simulink model "EE_Lab4"  (R2024b)
settings: Solver=VariableStepAuto  StartTime=0.0  StopTime=0.04  RelTol=1e-3
undefined symbols (not defined in the file): Angle, Magnitude
libraries: spsSeriesRLCBranchLib x4, spsCurrentMeasurementLib x4, spsVoltageMeasurementLib x4, spsACVoltageSourceLib x2, spsLinearTransformerLib x2, sps_lib x1, spspowerguiLib x1
settings Model: Creator=offic  LastModifiedBy=offic

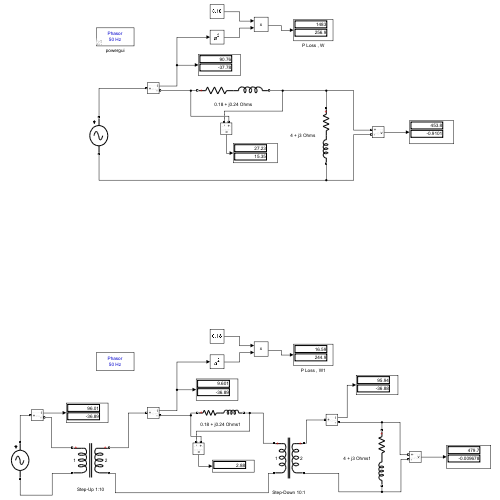
[thumbnail: Simulink's stored preview of the top-level diagram]
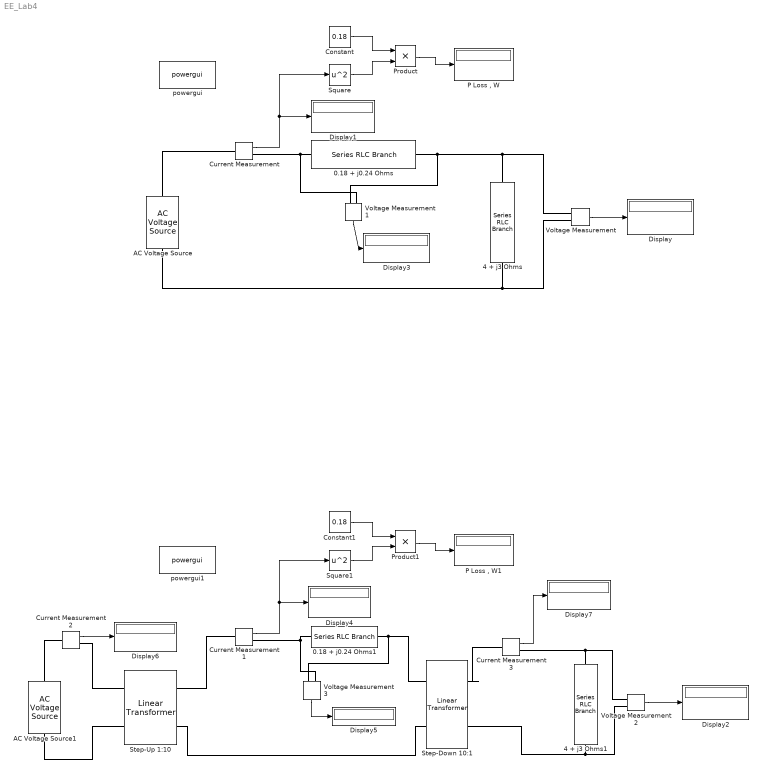
== system EE_Lab4 ==
  0.18 + j0.24 Ohms : spsSeriesRLCBranchLib/Series RLC Branch  LConnTagsString=__new0  RConnTagsString=__new0  BranchType=RL  Resistance=0.18  Inductance=0.0007639437  SetiL0=off  InitialCurrent=0  Capacitance=1e-6  Setx0=off  InitialVoltage=0  Measurements=None
  0.18 + j0.24 Ohms1 : spsSeriesRLCBranchLib/Series RLC Branch  LConnTagsString=__new0  RConnTagsString=__new0  BranchType=RL  Resistance=0.18  Inductance=0.0007639437  SetiL0=off  InitialCurrent=0  Capacitance=1e-6  Setx0=off  InitialVoltage=0  Measurements=None
  4 + j3 Ohms : spsSeriesRLCBranchLib/Series RLC Branch  LConnTagsString=__new0  RConnTagsString=__new0  BranchType=RL  Resistance=4  Inductance=0.00954929  SetiL0=off  InitialCurrent=0  Capacitance=1e-6  Setx0=off  InitialVoltage=0  Measurements=None
  4 + j3 Ohms1 : spsSeriesRLCBranchLib/Series RLC Branch  LConnTagsString=__new0  RConnTagsString=__new0  BranchType=RL  Resistance=4  Inductance=0.00954929  SetiL0=off  InitialCurrent=0  Capacitance=1e-6  Setx0=off  InitialVoltage=0  Measurements=None
  AC Voltage Source : spsACVoltageSourceLib/AC Voltage Source  Amplitude=480  Phase=0  Frequency=50  SampleTime=0  Measurements=None  BusType=swing  Pref=10e3  Qref=0  Qmin=-inf  Qmax=+inf
  AC Voltage Source1 : spsACVoltageSourceLib/AC Voltage Source  Amplitude=480  Phase=0  Frequency=50  SampleTime=0  Measurements=None  BusType=swing  Pref=10e3  Qref=0  Qmin=-inf  Qmax=+inf
  Constant : Constant  Value=0.18
  Constant1 : Constant  Value=0.18
  Current Measurement{,1..3} (4 alike) : spsCurrentMeasurementLib/Current Measurement  PhasorSimulation=on  OutputType=Magnitude-Angle  PSBequivalent=0
  Display{,1..7} (8 alike) : Display
  "P Loss , W" : Display
  "P Loss , W1" : Display
  Product : Product
  Product1 : Product
  Square : Math  Operator=square
  Square1 : Math  Operator=square
  Step-Down 10:1 : spsLinearTransformerLib/Linear Transformer  UNITS=SI  NominalPower=[ 250e6 50 ]  winding1="[ 4800  0.0000001  0.00000001]"  winding2="[ 480  0.0000001  0.00000001]"  ThreeWindings=off  winding3=[3.15e+05 0.7938 0.10107]  RmLm=[1.08e6 2866]  Measurements=None  DataType=on
  Step-Up 1:10 : spsLinearTransformerLib/Linear Transformer  UNITS=SI  NominalPower=[ 250e6 50 ]  winding1="[ 480  0.0000001  0.00000001]"  winding2="[ 4800  0.0000001  0.00000001]"  ThreeWindings=off  winding3=[3.15e+05 0.7938 0.10107]  RmLm=[1.08e6 2866]  Measurements=None  DataType=on
  Voltage Measurement : spsVoltageMeasurementLib/Voltage Measurement  PhasorSimulation=on  OutputType=Magnitude-Angle  PSBequivalent=0
  Voltage Measurement1 : spsVoltageMeasurementLib/Voltage Measurement  PhasorSimulation=on  OutputType=Magnitude-Angle  PSBequivalent=0
  Voltage Measurement2 : spsVoltageMeasurementLib/Voltage Measurement  PhasorSimulation=on  OutputType=Magnitude-Angle  PSBequivalent=0
  Voltage Measurement3 : spsVoltageMeasurementLib/Voltage Measurement  PhasorSimulation=on  OutputType=Magnitude  PSBequivalent=0
  powergui : sps_lib/powergui  Priority=1  SimulationMode=Phasor  SampleTime=50e-6  frequency=50  Iterations=50  frequencyindice=50  Pbase=100e6  ErrMax=1e-4  UnitsV=kV  UnitsW=MW  buscounter=0  FunctionMessages=off  echomessages=off  EnableUseOfTLC=off  CurrentSourceSwitches=off  DisableSnubberDevices=off  DisableRonSwitches=off  DisableVfSwitches=off  DisplayEquations=off  AutomaticDiscreteSolvers=off  SolverType=Tustin/Backward Euler (TBE)  Interpol=off  ExternalGateDelay=off  methode=off  Ts=100  x0status=blocks  SPID=on  SwTol=0  HookPort=off  NonlinearTolerance=1e-4  nMaxIteration=100  ContinueOnMaxIteration=off  RestoreLinks=warning  ResistiveCurrentMeasurement=off  Frange=[0:2:500]  Ylog=off  Xlog=on  ShowGrid=off  save=off  variable=ZData  structure=0  ZoomFFT=off  StartTime=0.0  cycles=1  DisplayStyle=1  fundamental=60  FreqAxis=off  MaxFrequency=1000  frequencyindicesteady=1  RmsSteady=1  display=off
  powergui1 : spspowerguiLib/powergui  Priority=1  SimulationMode=Phasor  SampleTime=50e-6  frequency=50  Iterations=50  frequencyindice=50  Pbase=100e6  ErrMax=1e-4  UnitsV=kV  UnitsW=MW  buscounter=0  FunctionMessages=off  echomessages=off  EnableUseOfTLC=off  CurrentSourceSwitches=off  DisableSnubberDevices=off  DisableRonSwitches=off  DisableVfSwitches=off  DisplayEquations=off  AutomaticDiscreteSolvers=off  SolverType=Tustin/Backward Euler (TBE)  Interpol=off  ExternalGateDelay=off  methode=off  Ts=100  x0status=blocks  SPID=on  SwTol=0  HookPort=off  NonlinearTolerance=1e-4  nMaxIteration=100  ContinueOnMaxIteration=off  RestoreLinks=warning  ResistiveCurrentMeasurement=off  Frange=[0:2:500]  Ylog=off  Xlog=on  ShowGrid=off  save=off  variable=ZData  structure=0  ZoomFFT=off  StartTime=0.0  cycles=1  DisplayStyle=1  fundamental=60  FreqAxis=off  MaxFrequency=1000  frequencyindicesteady=1  RmsSteady=1  display=off
  wires:
  Voltage Measurement/1 -> Display/1
  Current Measurement/1 -> Square/1, Display1/1
  Constant/1 -> Product/1
  Square/1 -> Product/2
  Product/1 -> "P Loss , W"/1
  Voltage Measurement1/1 -> Display3/1
  Voltage Measurement3/1 -> Display5/1
  Voltage Measurement2/1 -> Display2/1
  Square1/1 -> Product1/2
  Product1/1 -> "P Loss , W1"/1
  Constant1/1 -> Product1/1
  Current Measurement1/1 -> Square1/1, Display4/1
  Current Measurement2/1 -> Display6/1
  Current Measurement3/1 -> Display7/1
  connections:
  AC Voltage Source/RConn1 -- Current Measurement/LConn1
  0.18 + j0.24 Ohms/LConn1 -- Voltage Measurement1/LConn1 -- Current Measurement/RConn1
  0.18 + j0.24 Ohms/RConn1 -- Voltage Measurement1/LConn2 -- 4 + j3 Ohms/LConn1 -- Voltage Measurement/LConn1
  AC Voltage Source/LConn1 -- 4 + j3 Ohms/RConn1 -- Voltage Measurement/LConn2
  0.18 + j0.24 Ohms1/RConn1 -- Voltage Measurement3/LConn2 -- Step-Down 10:1/LConn1
  Voltage Measurement2/LConn2 -- Step-Down 10:1/RConn2 -- 4 + j3 Ohms1/RConn1
  0.18 + j0.24 Ohms1/LConn1 -- Voltage Measurement3/LConn1 -- Current Measurement1/RConn1
  AC Voltage Source1/LConn1 -- Step-Up 1:10/LConn2
  AC Voltage Source1/RConn1 -- Current Measurement2/LConn1
  Current Measurement2/RConn1 -- Step-Up 1:10/LConn1
  Step-Up 1:10/RConn1 -- Current Measurement1/LConn1
  Voltage Measurement2/LConn1 -- 4 + j3 Ohms1/LConn1 -- Current Measurement3/RConn1
  Step-Down 10:1/RConn1 -- Current Measurement3/LConn1
  Step-Up 1:10/RConn2 -- Step-Down 10:1/LConn2
